simulink model "regulator_LQG_discrete_Ueq"  (R2019b)
settings: Solver=ode45  StartTime=0.0  StopTime=tsim  RelTol=1e-3  EnableMultiTasking=on
values from neighbouring files (symbols this model uses):
  B_noise = [B ones(size(B,1),1)]    [es3.m]
  C_states = eye(2)    [es3.m]
  D_noise = [D_states zeros(size(D_states,1),1)]    [es3.m]
  Klqr1 = dlqr(A,B,Q,R)    [es3.m]
  NK = 0    [es3.m]
  RK = QK(1)*0.1    [es3.m]
  sat_max = inf    [es3.m]
  sat_min = -inf    [es3.m]
  Ts = 0.1    [es3.m]
  Ubar = inv(dcgain(Gz))*Ybar    [es3.m]
  x0 = [5 20]    [es3.m]
  x0K = 1.5*x0    [es3.m]
  xref = Xbar    [es3.m]
undefined symbols (not defined in the file or in its folder): A, B, C, D, Discrete, Time
libraries: simulink x2, ctrlSharedLib x1
settings Model: Creator=Administrator  LastModifiedBy=Chiara
settings DataIOCC: LimitDataPoints=on  SaveFormat=Array  SignalLoggingSaveFormat=ModelDataLogs  ReturnWorkspaceOutputs=off
settings OptimizationCC: ExpressionDepthLimit=2147483647  InitFltsAndDblsToZero=on  LifeSpan=inf
settings DebuggingCC: UnderspecifiedInitializationDetection=Classic  MergeDetectMultiDrivingBlocksExec=none  SolverPrmCheckMsg=warning  FcnCallInpInsideContextMsg=warning  StateNameClashWarn=warning  SFUnexpectedBacktrackingDiag=warning  SFNoUnconditionalDefaultTransitionDiag=warning  SFExecutionAtInitializationDiag=none  ArithmeticOperatorsInVariantConditions=warning
settings HardwareCC: ProdBitPerPointer=32  ProdBitPerSizeT=32  ProdBitPerPtrDiffT=32  ProdLargestAtomicFloat=None  ProdIntDivRoundTo=Undefined  ProdEndianess=Unspecified  ProdWordSize=32  ProdHWDeviceType=32-bit Generic
settings ModelReferenceCC: PropagateSignalLabelsOutOfModel=off
settings SFSimCC: SimUseLocalCustomCode=off  CustomCodeUndefinedFunction=UseInterfaceOnly
settings RTWCC: RTWUseLocalCustomCode=off
settings CodeAppCC: StateflowObjectComments=on
settings GRTTargetCC: TargetLangStandard=C89/C90 (ANSI)  GeneratePreprocessorConditionals=Disable all  CombineOutputUpdateFcns=off  GRTInterface=on
settings ConfigComp: CovMetricSettings=dw  CovHtmlReporting=on  CovSaveCumulativeToWorkspaceVar=on  CovSaveSingleToWorkspaceVar=on  CovExternalEMLEnable=off  CovSFcnEnable=off

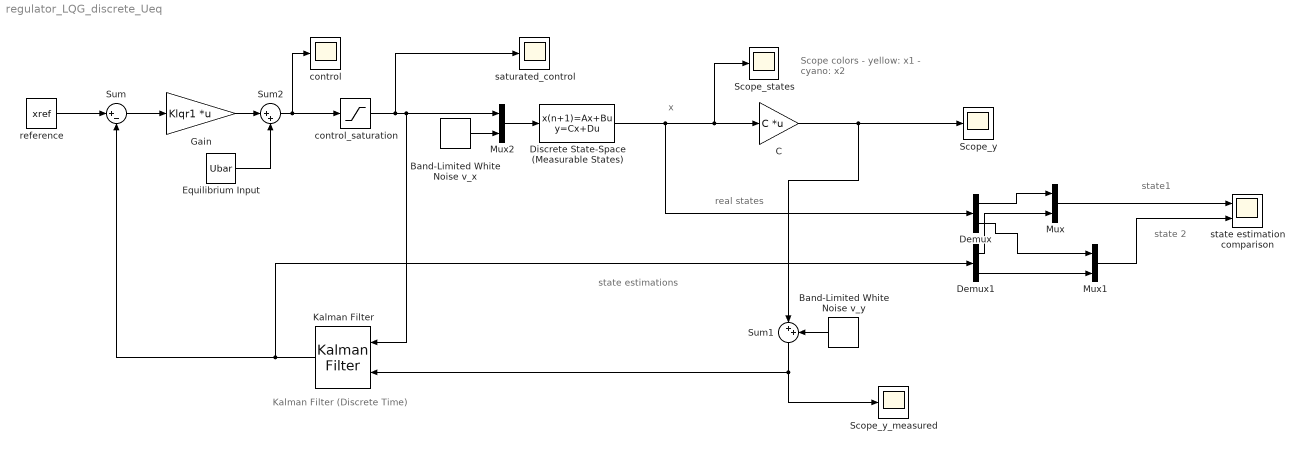
== system regulator_LQG_discrete_Ueq ==
  note: Kalman Filter (Discrete Time)
  note: state 2
  note: state1
  note: real states
  note: state estimations
  note: x
  note: Scope colors
      | - yellow: x1
      | - cyano: x2
  "Band-Limited White Noise v_x " : simulink/Sources/Band-Limited White Noise  Cov=power_vx  Ts=Ts  seed=[23341]
  Band-Limited White Noise v_y : simulink/Sources/Band-Limited White Noise  Cov=power_vy  Ts=Ts  seed=[1258]
  C : Gain  Gain=C  Multiplication=Matrix(K*u)
  Demux : Demux  Outputs=2
  Demux1 : Demux  Outputs=2
  "Discrete State-Space (Measurable States) " : DiscreteStateSpace  A=A  B=B_noise  C=C_states  D=D_noise  InitialCondition=x0  SampleTime=Ts
  Equilibrium Input : Constant  Value=Ubar
  Gain : Gain  Gain=Klqr1  Multiplication=Matrix(K*u)
  Kalman Filter : ctrlSharedLib/Kalman Filter  TimeDomain=Discrete-Time  UseCurrentEstimator=on  ModelSource=Individual A, B, C, D matrices  ModelSourceVariable=ss(0.95,1,1,0,1)  A=A  B=B  C=C  D=D  NumberOfStates=1  NumberOfInputs=1  NumberOfOutputs=1  InitialEstimateSource=Dialog  X0=x0K  P0=10  UseK=off  UseGH=off  NumberOfProcessNoiseInputs=1  G=1  TimeInvariantG=on  H=0  TimeInvariantH=on  Q=QK  TimeInvariantQ=on  R=RK  TimeInvariantR=on  N=NK  TimeInvariantN=on  AddInputPort=on  AddEnablePort=off  OutputEstimatedY=off  OutputP=off  Ts=Ts
      settings: SourceProductBaseCode=CT
  Mux : Mux  Inputs=2
  Mux1 : Mux  Inputs=2
  Mux2 : Mux  Inputs=2
  Scope_states : Scope
  Scope_y : Scope
  Scope_y_measured : Scope
  Sum : Sum  Inputs=|+-
  Sum1 : Sum  Inputs=|++
  Sum2 : Sum  Inputs=|++
  control : Scope
  control_saturation : Saturate  UpperLimit=sat_max  LowerLimit=sat_min
  reference : Constant  Value=xref
  saturated_control : Scope
  "state estimation comparison " : Scope  NumInputPorts=2
  wires:
  reference/1 -> Sum/1
  Sum/1 -> Gain/1
  "Discrete State-Space (Measurable States) "/1 -> Demux/1, Scope_states/1, C/1
  C/1 -> Sum1/1, Scope_y/1
  control_saturation/1 -> Mux2/1, Kalman Filter/1, saturated_control/1
  Kalman Filter/1 -> Demux1/1, Sum/2
  Demux/1 -> Mux/1
  Demux1/1 -> Mux/2
  Demux1/2 -> Mux1/2
  Demux/2 -> Mux1/1
  Mux1/1 -> "state estimation comparison "/2
  Mux/1 -> "state estimation comparison "/1
  Mux2/1 -> "Discrete State-Space (Measurable States) "/1
  Sum1/1 -> Scope_y_measured/1, Kalman Filter/2
  Band-Limited White Noise v_y/1 -> Sum1/2
  "Band-Limited White Noise v_x "/1 -> Mux2/2
  Gain/1 -> Sum2/1
  Sum2/1 -> control/1, control_saturation/1
  Equilibrium Input/1 -> Sum2/2
